simulink model "sampleModel1787_sub_sub_sub"  (R2023a)
settings: Solver=VariableStepAuto  StartTime=0.0  StopTime=10.0  RelTol=1e-3
libraries: hdlsllib x3, simulink x3
settings Model: Creator=user1  LastModifiedBy=user1
settings OptimizationCC: BlockReduction=off  ConditionallyExecuteInputs=off

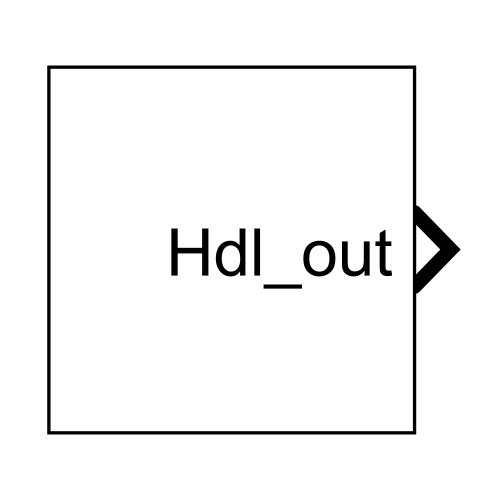
[thumbnail: Simulink's stored preview of the top-level diagram]
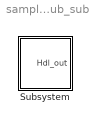
== system sampleModel1787_sub_sub_sub ==
  Subsystem : Subsystem

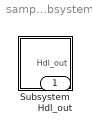
== system sampleModel1787_sub_sub_sub/Subsystem ==
  Subsystem : Subsystem
  Hdl_out : Outport  OutDataTypeStr=uint8

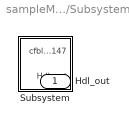
== system sampleModel1787_sub_sub_sub/Subsystem/Subsystem ==
  Subsystem : Subsystem
  Hdl_out : Outport  OutDataTypeStr=uint8

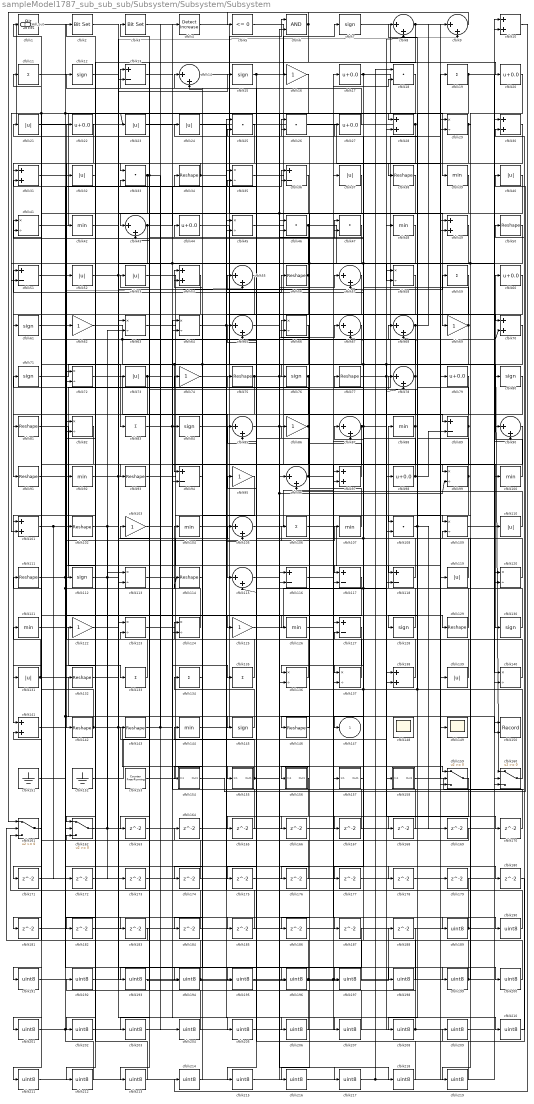
== system sampleModel1787_sub_sub_sub/Subsystem/Subsystem/Subsystem ==
  cfblk1 : hdlsllib/Logic and Bit Operations/Bit Shift  mode=Shift Left Logical  N=0
  cfblk{10,28,30..31,49,54,70,97,101,138,141} (11 alike) : Sum  OutDataTypeStr=uint8
  cfblk{39,42,48,88,92,100,104,107,121,126,144} (11 alike) : MinMax  OutDataTypeStr=uint8
  cfblk{34,38,50,56,75,77,81,91,93,102,111,114,129,132,142..143,146} (17 alike) : Reshape
  cfblk{16,62,69,74,86,95,103,122,125} (9 alike) : Gain  OutDataTypeStr=uint8
  cfblk{8..9,14,43,55,57,65,67..68,78,85,87,90,96,105,115} (16 alike) : Sum  Inputs=|++  OutDataTypeStr=uint8
  cfblk{11,19,59,83,106,133..135} (8 alike) : Sum  Inputs=+  OutDataTypeStr=uint8
  cfblk{18,25..26,33,46..47,108} (7 alike) : DotProduct  OutDataTypeStr=uint8
  cfblk{29,35,41,45,58,63..64,66,72,82,99,109,113,120,123..124,136..137,140} (19 alike) : Product  Inputs=*/  OutDataTypeStr=uint8  RndMeth=Zero  SaturateOnIntegerOverflow=on
  cfblk{21,23..24,32,37,40,52..53,73,110,119,131,139} (13 alike) : Abs  OutDataTypeStr=uint8  SaturateOnIntegerOverflow=off
  cfblk{7,12,15,61,71,76,80,84,112,128,130,145} (12 alike) : Signum
  cfblk{13,36,51,89,94,116..118,127} (9 alike) : Sum  Inputs=+-  OutDataTypeStr=uint8
  cfblk148 : Scope
      settings: Floating=on
  cfblk149 : Scope
  cfblk150 : Record  FileSettingsInternal="{\"entries\":[{\"content\":{\"excelSettings\":{\"content\":{},\"type\":\"Streamout.ExcelSettings\"}},\"type\":\"Streamout.FileSettingStorage\",\"uuid\":\"\"}],\"packageUris\":[\"http:\\/\\/schema.mathworks.com\\/mf0\\/streamout_blocks\\/R2020a\"],\"version\":\"1.0\"}"  Layout=[1 1]  SignalsInternal="{\"entries\":[{\"content\":{\"signals\":[{\"content\":{\"blockPath\":[],\"dimensions\":[1],\"domain\":\"\",\"lineColor\":\"#a2142f\",\"plots\":[1],\"port\":1,\"signalID\":42478,\"signalName\":\"cfblk194\"},\"type\":\"RecordBlkView.Signal\",\"uuid\":\"\"},{\"content\":{\"blockPath\":[],\"dimensions\":[1],\"domain\":\"\",\"lineColor\":\"#139fff\",\"plots\":[1],\"port\":2,\"signalID\":42481,\"signalName\":\"cfblk51\"},\"type\":\"RecordBlkView.Signal\",\"uuid\":\"\"}]},\"type\":\"RecordBlkView.InputSignals\",\"uuid\":\"\"}],\"packageUris\":[\"http:\\/\\/schema.mathworks.com\\/mf0\\/streamout_blocks\\/R2020a\"],\"version\":\"1.0\"}"  VisualizationBindings="{\"xyplotplugin\":{\"info\":[{\"series\":[{\"bindingParametersList\":[{\"parameter\":\"X-Axis\",\"signalID\":42478,\"signalName\":\"cfblk194\"},{\"parameter\":\"Y-Axis\",\"signalID\":42481,\"signalName\":\"cfblk51\"}],\"seriesID\":11564}],\"subplotID\":1}]}}"  CompatibilityTag=XY  st=-1
  cfblk151 : Ground
  cfblk152 : Ground
  cfblk153 : hdlsllib/Sources/Counter Free-Running  NumBits=16  tsamp=-1
  cfblk154 : Subsystem
      settings: LibrarySourceBlock=|
      | hdlsllib/Ports &
      | Subsystems/Subsystem
  cfblk155 : Subsystem
      settings: LibrarySourceBlock=|
      | hdlsllib/Ports &
      | Subsystems/Subsystem
  cfblk156 : Subsystem
      settings: LibrarySourceBlock=|
      | hdlsllib/Ports &
      | Subsystems/Subsystem
  cfblk157 : Subsystem
      settings: LibrarySourceBlock=|
      | hdlsllib/Ports &
      | Subsystems/Subsystem
  cfblk158 : Subsystem
      settings: LibrarySourceBlock=|
      | hdlsllib/Ports &
      | Subsystems/Subsystem
  cfblk{159..162} (4 alike) : Switch  OutDataTypeStr=uint8  SaturateOnIntegerOverflow=off  InputSameDT=off
  cfblk{163..188} (26 alike) : Delay  SampleTime=1
  cfblk{17,20,22,27,44,60,79,98} (8 alike) : Bias  Bias=0.0  SaturateOnIntegerOverflow=off
  cfblk{189..219} (31 alike) : DataTypeConversion  OutDataTypeStr=uint8  SaturateOnIntegerOverflow=off  RndMeth=Floor
  cfblk2 : simulink/Logic and Bit Operations/Bit Set  iBit=0
      settings: LibrarySourceBlock=|
      | hdlsllib/Logic and Bit
      | Operations/Bit Set
  cfblk3 : simulink/Logic and Bit Operations/Bit Set  iBit=0
      settings: LibrarySourceBlock=|
      | hdlsllib/Logic and Bit
      | Operations/Bit Set
  cfblk4 : simulink/Logic and Bit Operations/Detect Increase  vinit=0.0  OutDataTypeStr=uint8
      settings: LibrarySourceBlock=|
      | hdlsllib/Logic and Bit
      | Operations/Detect
      | Increase
  cfblk5 : hdlsllib/Logic and Bit Operations/Compare To Zero  relop=<=  OutDataTypeStr=uint8
  cfblk6 : Logic  AllPortsSameDT=off  OutDataTypeStr=boolean
  cfblk147 : Outport  OutDataTypeStr=uint8  VectorParamsAs1DForOutWhenUnconnected=off
  Hdl_out : Outport  Port=2  OutDataTypeStr=uint8
  wires:
  cfblk101/1 -> cfblk172/1, cfblk138/2
  cfblk67/1 -> cfblk83/1
  cfblk119/1 -> cfblk24/1
  cfblk41/1 -> cfblk39/1
  cfblk32/1 -> cfblk141/1
  cfblk144/1 -> cfblk6/1
  cfblk22/1 -> cfblk142/1
  cfblk46/1 -> cfblk163/1, cfblk140/1
  cfblk115/1 -> cfblk99/2, cfblk57/1
  cfblk111/1 -> cfblk129/1, cfblk75/1
  cfblk4/1 -> cfblk28/1
  cfblk35/1 -> cfblk89/1
  cfblk128/1 -> cfblk88/1
  cfblk118/1 -> cfblk13/1
  cfblk53/1 -> cfblk117/1
  cfblk98/1 -> cfblk51/1, cfblk89/2
  cfblk124/1 -> cfblk104/1
  cfblk60/1 -> cfblk91/1
  cfblk27/1 -> cfblk12/1
  cfblk63/1 -> cfblk108/1
  cfblk64/1 -> cfblk56/1, cfblk78/2, cfblk160/1
  cfblk133/1 -> cfblk22/1
  cfblk76/1 -> cfblk84/1, cfblk156/1(In1)
  cfblk1/1 -> cfblk52/1
  cfblk5/1 -> cfblk158/1(In1)
  cfblk102/1 -> cfblk173/1, cfblk13/2
  cfblk85/1 -> cfblk47/1, cfblk130/1
  cfblk121/1 -> cfblk133/1
  cfblk57/1 -> cfblk136/1
  cfblk112/1 -> cfblk105/1, cfblk113/1
  cfblk68/1 -> cfblk9/1, cfblk72/2, cfblk94/1
  cfblk14/1 -> cfblk69/1
  cfblk48/1 -> cfblk176/1, cfblk137/1
  cfblk123/1 -> cfblk19/1
  cfblk160/1 -> cfblk78/1, cfblk67/2, cfblk86/1
  cfblk29/1 -> cfblk219/1, cfblk61/1
  cfblk139/1 -> cfblk54/1
  cfblk51/1 -> cfblk185/1, cfblk150/2
  cfblk66/1 -> cfblk93/1
  cfblk120/1 -> cfblk47/2, cfblk62/1
  cfblk6/1 -> cfblk132/1, cfblk161/1
  cfblk11/1 -> cfblk55/2, cfblk23/1
  cfblk44/1 -> cfblk119/1
  cfblk56/1 -> cfblk184/1, cfblk21/1
  cfblk125/1 -> cfblk28/2
  cfblk17/1 -> cfblk57/2, cfblk79/1
  cfblk152/1 -> cfblk98/1
  cfblk15/1 -> cfblk115/2, cfblk7/1
  cfblk59/1 -> cfblk146/1
  cfblk105/1 -> cfblk37/1
  cfblk116/1 -> cfblk189/1
  cfblk62/1 -> cfblk70/2, cfblk76/1
  cfblk81/1 -> cfblk118/1
  cfblk104/1 -> cfblk58/1
  cfblk25/1 -> cfblk131/1
  cfblk157/1(Out1) -> cfblk87/1
  cfblk158/1(Out1) -> cfblk50/1
  cfblk87/1 -> cfblk137/2, cfblk170/1, cfblk27/1
  cfblk151/1 -> cfblk42/1
  cfblk153/1 -> cfblk16/1
  cfblk16/1 -> cfblk101/2, cfblk31/1
  cfblk99/1 -> cfblk8/1, cfblk128/1
  cfblk34/1 -> cfblk105/2, cfblk33/1
  cfblk142/1 -> cfblk71/1, cfblk9/2, cfblk155/1(In1)
  cfblk72/1 -> cfblk115/1
  cfblk33/1 -> cfblk113/2, cfblk204/1, cfblk203/1
  cfblk122/1 -> cfblk199/1
  cfblk154/1(Out1) -> cfblk40/1
  cfblk37/1 -> cfblk126/1
  cfblk106/1 -> cfblk139/1
  cfblk114/1 -> cfblk74/1
  cfblk18/1 -> cfblk136/2
  cfblk55/1 -> cfblk92/1
  cfblk7/1 -> cfblk20/1
  cfblk43/1 -> cfblk36/2, cfblk112/1
  cfblk141/1 -> cfblk114/1, cfblk106/1
  cfblk40/1 -> cfblk43/1
  cfblk162/1 -> cfblk63/2, cfblk118/2
  cfblk145/1 -> cfblk124/1
  cfblk89/1 -> cfblk125/1, cfblk25/2
  cfblk9/1 -> cfblk5/1
  cfblk26/1 -> cfblk49/1
  cfblk131/1 -> cfblk157/1(In1), cfblk121/1
  cfblk137/1 -> cfblk14/1
  cfblk155/1(Out1) -> cfblk187/1, cfblk144/1
  cfblk65/1 -> cfblk217/1
  cfblk77/1 -> cfblk8/2, cfblk100/1
  cfblk135/1 -> cfblk14/2
  cfblk100/1 -> cfblk60/1
  cfblk42/1 -> cfblk36/1
  cfblk93/1 -> cfblk149/1
  cfblk12/1 -> cfblk45/2
  cfblk80/1 -> cfblk81/1
  cfblk30/1 -> cfblk208/1
  cfblk129/1 -> cfblk26/1
  cfblk47/1 -> cfblk186/1, cfblk51/2, cfblk94/2
  cfblk143/1 -> cfblk4/1, cfblk145/1
  cfblk109/1 -> cfblk80/1
  cfblk103/1 -> cfblk159/1
  cfblk94/1 -> cfblk44/1
  cfblk92/1 -> cfblk124/2, cfblk59/1
  cfblk24/1 -> cfblk70/1
  cfblk75/1 -> cfblk212/1, cfblk218/1, cfblk67/1
  cfblk107/1 -> cfblk55/1
  cfblk70/1 -> cfblk147/1, cfblk202/1, cfblk174/1
  cfblk108/1 -> cfblk169/1, cfblk168/1, cfblk68/2
  cfblk113/1 -> cfblk107/1
  cfblk127/1 -> cfblk196/1
  cfblk83/1 -> cfblk68/1, cfblk117/2
  cfblk90/1 -> cfblk201/1
  cfblk19/1 -> cfblk38/1, cfblk110/1
  cfblk49/1 -> cfblk159/2
  cfblk110/1 -> cfblk96/2
  cfblk91/1 -> cfblk35/2
  cfblk97/1 -> cfblk26/2
  cfblk95/1 -> cfblk194/1
  cfblk138/1 -> cfblk53/1
  cfblk69/1 -> cfblk41/2, cfblk101/1
  cfblk71/1 -> cfblk73/1
  cfblk45/1 -> cfblk138/1
  cfblk140/1 -> cfblk85/2
  cfblk28/1 -> Hdl_out/1, cfblk32/1
  cfblk8/1 -> cfblk43/2, cfblk29/2
  cfblk73/1 -> cfblk135/1, cfblk162/1
  cfblk134/1 -> cfblk154/1(In1)
  cfblk50/1 -> cfblk175/1, cfblk99/1
  cfblk13/1 -> cfblk97/2
  cfblk130/1 -> cfblk72/1, cfblk77/1
  cfblk78/1 -> cfblk162/2, cfblk41/1
  cfblk96/1 -> cfblk18/2, cfblk31/2
  cfblk146/1 -> cfblk66/1
  cfblk36/1 -> cfblk181/1, cfblk66/2
  cfblk86/1 -> cfblk182/1, cfblk11/1
  cfblk88/1 -> cfblk177/1, cfblk33/2
  cfblk136/1 -> cfblk34/1
  cfblk20/1 -> cfblk109/1
  cfblk132/1 -> cfblk15/1
  cfblk52/1 -> cfblk195/1, cfblk58/2
  cfblk54/1 -> cfblk64/2
  cfblk163/1 -> cfblk96/1
  cfblk164/1 -> cfblk46/2
  cfblk156/1(Out1) -> cfblk165/1
  cfblk165/1 -> cfblk25/1
  cfblk58/1 -> cfblk166/1
  cfblk166/1 -> cfblk120/1
  cfblk39/1 -> cfblk167/1
  cfblk167/1 -> cfblk64/1
  cfblk168/1 -> cfblk85/1
  cfblk169/1 -> cfblk162/3
  cfblk170/1 -> cfblk54/2
  cfblk117/1 -> cfblk171/1
  cfblk171/1 -> cfblk45/1
  cfblk173/1 -> cfblk6/2
  cfblk174/1 -> cfblk63/1
  cfblk175/1 -> cfblk160/2
  cfblk176/1 -> cfblk141/2
  cfblk177/1 -> cfblk108/2
  cfblk61/1 -> cfblk178/1
  cfblk178/1 -> cfblk29/1
  cfblk179/1 -> cfblk161/3
  cfblk126/1 -> cfblk180/1
  cfblk181/1 -> cfblk160/3
  cfblk21/1 -> cfblk183/1
  cfblk183/1 -> cfblk161/2
  cfblk184/1 -> cfblk1/1
  cfblk185/1 -> cfblk35/1
  cfblk186/1 -> cfblk140/2
  cfblk189/1 -> cfblk97/1, cfblk120/2
  cfblk172/1 -> cfblk190/1
  cfblk190/1 -> cfblk116/1
  cfblk161/1 -> cfblk191/1
  cfblk191/1 -> cfblk116/2
  cfblk188/1 -> cfblk192/1
  cfblk192/1 -> cfblk123/1
  cfblk38/1 -> cfblk193/1
  cfblk193/1 -> cfblk188/1
  cfblk194/1 -> cfblk123/2, cfblk17/1, cfblk150/1
  cfblk195/1 -> cfblk95/1
  cfblk196/1 -> cfblk111/1, cfblk49/2
  cfblk31/1 -> cfblk197/1
  cfblk197/1 -> cfblk127/1
  cfblk182/1 -> cfblk198/1
  cfblk198/1 -> cfblk127/2
  cfblk199/1 -> cfblk134/1, cfblk109/2
  cfblk23/1 -> cfblk200/1
  cfblk200/1 -> cfblk122/1
  cfblk201/1 -> cfblk87/2, cfblk102/1
  cfblk202/1 -> cfblk90/1
  cfblk203/1 -> cfblk90/2
  cfblk204/1 -> cfblk2/1
  cfblk2/1 -> cfblk205/1
  cfblk205/1 -> cfblk48/1
  cfblk74/1 -> cfblk206/1
  cfblk206/1 -> cfblk3/1
  cfblk3/1 -> cfblk207/1
  cfblk207/1 -> cfblk103/1
  cfblk208/1 -> cfblk143/1, cfblk159/3
  cfblk180/1 -> cfblk209/1
  cfblk209/1 -> cfblk30/1
  cfblk84/1 -> cfblk210/1
  cfblk210/1 -> cfblk30/2
  cfblk82/1 -> cfblk211/1
  cfblk211/1 -> cfblk46/1
  cfblk212/1 -> cfblk82/1
  cfblk187/1 -> cfblk213/1
  cfblk213/1 -> cfblk82/2
  cfblk10/1 -> cfblk214/1
  cfblk214/1 -> cfblk164/1
  cfblk79/1 -> cfblk215/1
  cfblk215/1 -> cfblk10/1
  cfblk159/1 -> cfblk216/1
  cfblk216/1 -> cfblk10/2
  cfblk217/1 -> cfblk18/1, cfblk179/1
  cfblk218/1 -> cfblk65/1
  cfblk219/1 -> cfblk65/2

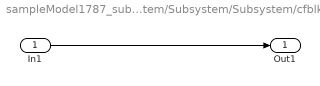
== system sampleModel1787_sub_sub_sub/Subsystem/Subsystem/Subsystem/cfblk154 ==
  In1 : Inport
  Out1 : Outport
  wires:
  In1/1 -> Out1/1

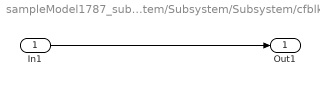
== system sampleModel1787_sub_sub_sub/Subsystem/Subsystem/Subsystem/cfblk155 ==
  In1 : Inport
  Out1 : Outport
  wires:
  In1/1 -> Out1/1

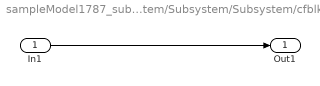
== system sampleModel1787_sub_sub_sub/Subsystem/Subsystem/Subsystem/cfblk156 ==
  In1 : Inport
  Out1 : Outport
  wires:
  In1/1 -> Out1/1

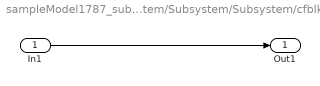
== system sampleModel1787_sub_sub_sub/Subsystem/Subsystem/Subsystem/cfblk157 ==
  In1 : Inport
  Out1 : Outport
  wires:
  In1/1 -> Out1/1

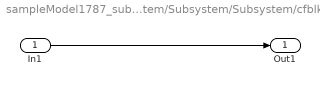
== system sampleModel1787_sub_sub_sub/Subsystem/Subsystem/Subsystem/cfblk158 ==
  In1 : Inport
  Out1 : Outport
  wires:
  In1/1 -> Out1/1
